simulink model "slotted_beam"  (R2024b)
settings: Solver=VariableStepAuto  StartTime=0.0  StopTime=10.0  RelTol=1e-3
settings Model: Creator=aldis  LastModifiedBy=aldis

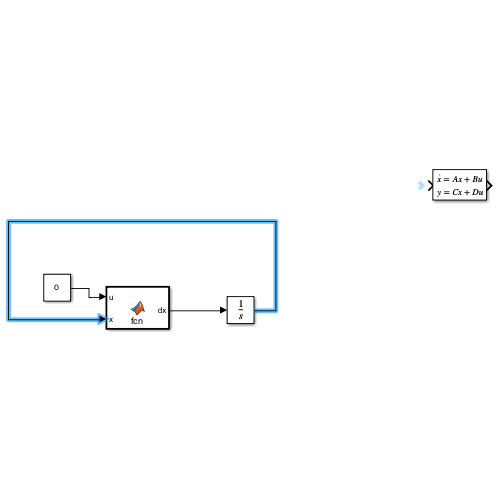
[thumbnail: Simulink's stored preview of the top-level diagram]
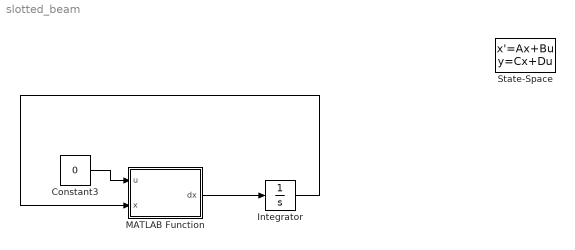
== system slotted_beam ==
  Constant3 : Constant  Value=0
  Integrator : Integrator  InitialCondition=[0;0;0;0]
  MATLAB Function : MATLAB Function  TreatAsAtomicUnit=on
  State-Space : StateSpace  InitialCondition=0
  wires:
  MATLAB Function/1(dx) -> Integrator/1
  Integrator/1 -> MATLAB Function/2(x)
  Constant3/1 -> MATLAB Function/1(u)

== matlab function slotted_beam/MATLAB Function ==
  data: u input; dx output; x input
function dx = fcn(u, x)

x1=x(1);
x2=x(2);
x3=x(3);
x4=x(4);

g=9.81;
m=1;
Jb=1;
J=1;
r=1;
b=m/(m+Jb/(r^2));

dx =[x2;
    b*(x1*x4*x4-g*sin(x3));
    x4;
    (u-m*g*x1*cos(x3)-2*m*x1*x2*x4)/(m*x1*x1+J+Jb)];

end
